simulink model "DroneControl"  (R2020a)
settings: Solver=FixedStepDiscrete  StartTime=0.0  StopTime=10.0  FixedStep=1  MaxStep=1  RelTol=1e-3
values from neighbouring files (symbols this model uses):
  ts = 0.01    [SetWorkspace.m]    (also in signal.m = 0.1)
settings Model: Creator=robyr  LastModifiedBy=robyr
settings DataIOCC: ReturnWorkspaceOutputs=off

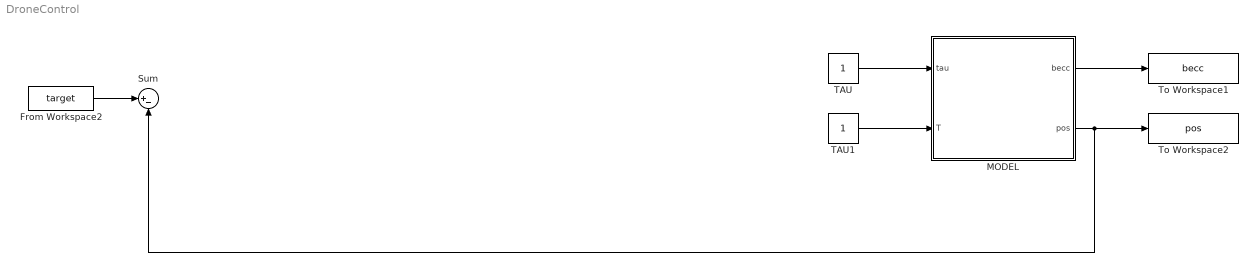
== system DroneControl ==
  From Workspace2 : FromWorkspace  VariableName=target  SampleTime=ts
  MODEL : Subsystem
  Sum : Sum  Inputs=|+-
  TAU : Constant
  TAU1 : Constant
  To Workspace1 : ToWorkspace  VariableName=becc  SampleTime=ts
  To Workspace2 : ToWorkspace  VariableName=pos  SampleTime=ts
  wires:
  From Workspace2/1 -> Sum/1
  MODEL/2(pos) -> To Workspace2/1, Sum/2
  TAU/1 -> MODEL/1(tau)
  TAU1/1 -> MODEL/2(T)
  MODEL/1(becc) -> To Workspace1/1

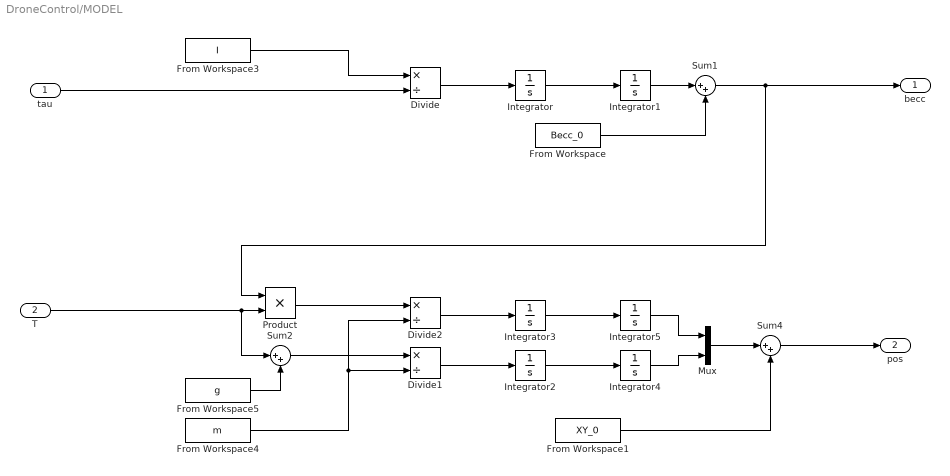
== system DroneControl/MODEL ==
  tau : Inport
  T : Inport  Port=2
  Divide : Product  Inputs=*/
  Divide1 : Product  Inputs=*/
  Divide2 : Product  Inputs=*/
  From Workspace : FromWorkspace  VariableName=Becc_0  SampleTime=ts
  From Workspace1 : FromWorkspace  VariableName=XY_0  SampleTime=ts
  From Workspace3 : FromWorkspace  VariableName=I  SampleTime=ts
  From Workspace4 : FromWorkspace  VariableName=m  SampleTime=ts
  From Workspace5 : FromWorkspace  VariableName=g  SampleTime=ts
  Integrator{,1..5} (6 alike) : Integrator
  Mux : Mux  Inputs=2
  Product : Product
  Sum1 : Sum  Inputs=|++
  Sum2 : Sum  Inputs=|++
  Sum4 : Sum  Inputs=|++
  becc : Outport
  pos : Outport  Port=2
  wires:
  Sum1/1 -> becc/1, Product/1
  Integrator2/1 -> Integrator4/1
  T/1 -> Sum2/1, Product/2
  Integrator/1 -> Integrator1/1
  From Workspace1/1 -> Sum4/2
  Mux/1 -> Sum4/1
  Integrator3/1 -> Integrator5/1
  Integrator5/1 -> Mux/1
  Integrator1/1 -> Sum1/1
  From Workspace3/1 -> Divide/1
  Integrator4/1 -> Mux/2
  Divide1/1 -> Integrator2/1
  From Workspace4/1 -> Divide2/2, Divide1/2
  tau/1 -> Divide/2
  Divide2/1 -> Integrator3/1
  Sum2/1 -> Divide1/1
  Product/1 -> Divide2/1
  From Workspace/1 -> Sum1/2
  From Workspace5/1 -> Sum2/2
  Divide/1 -> Integrator/1
  Sum4/1 -> pos/1
